simulink subsystem "queue_populator_model"  (R2020b)
settings: Solver=VariableStepAuto  StartTime=0.0  StopTime=10.0  RelTol=1e-3
undefined symbols (not defined in the file): kConsecutiveIndexDelta, kContainerIndexVector, kContainerLength, kFirstContainerIndex
libraries: move_index_lib x1
settings Model: Creator=rsub  LastModifiedBy=rsub

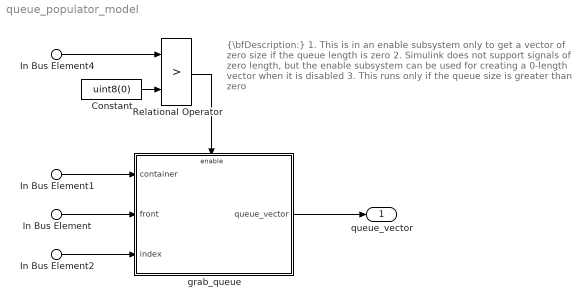
== system queue_populator_model ==
  note: {\bfDescription:}
      | 1. This is in an enable subsystem only to get a vector of zero size if the queue length is zero
      | 2. Simulink does not support signals of zero length, but the enable subsystem can be used for
      | creating a 0-length vector when it is disabled
      | 3. This runs only if the queue size is greater than zero
  In Bus Element : Inport  PortName=update_func_tx_bus  Element=front_index
  In Bus Element1 : Inport  PortName=update_func_tx_bus  Element=container_vector
  In Bus Element2 : Inport  PortName=update_func_tx_bus  Element=back_index
  In Bus Element4 : Inport  PortName=update_func_tx_bus  Element=queue_size
  Constant : Constant  Value=uint8(0)
  Relational Operator : RelationalOperator  Operator=>  OutDataTypeStr=boolean  RndMeth=Simplest
  grab_queue : Subsystem
  queue_vector : Outport
  wires:
  In Bus Element1/1 -> grab_queue/1(container)
  In Bus Element/1 -> grab_queue/2(front)
  In Bus Element2/1 -> grab_queue/3(index)
  grab_queue/1(queue_vector) -> queue_vector/1
  In Bus Element4/1 -> Relational Operator/1
  Relational Operator/1 -> grab_queue/Enable
  Constant/1 -> Relational Operator/2

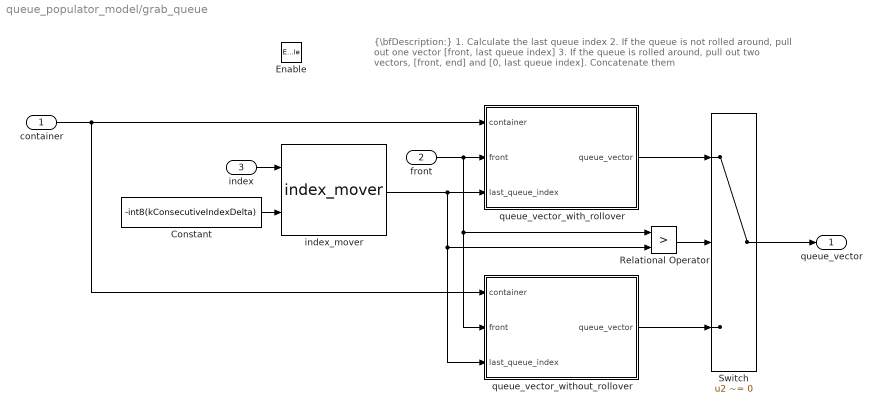
== system queue_populator_model/grab_queue ==
  note: {\bfDescription:}
      | 1. Calculate the last queue index
      | 2. If the queue is not rolled around, pull out one vector [front, last queue index]
      | 3. If the queue is rolled around, pull out two vectors, [front, end] and [0, last queue index]. Concatenate them
  container : Inport
  front : Inport  Port=2
  index : Inport  Port=3
  Enable : EnablePort  StatesWhenEnabling=reset  PropagateVarSize=During execution
  Constant : Constant  Value=-int8(kConsecutiveIndexDelta)
  Relational Operator : RelationalOperator  Operator=>  OutDataTypeStr=boolean  RndMeth=Simplest
  Switch : Switch  Criteria=u2 ~= 0  AllowDiffInputSizes=on
  index_mover : move_index_lib/index_mover  SystemSampleTime=-1  VariantActivationTime=update diagram  Latency=0  AutoFrameSizeCalculation=off
  queue_vector_with_rollover : Subsystem
  queue_vector_without_rollover : Subsystem
  queue_vector : Outport  OutputWhenDisabled=reset
  wires:
  queue_vector_with_rollover/1(queue_vector) -> Switch/1
  queue_vector_without_rollover/1(queue_vector) -> Switch/3
  container/1 -> queue_vector_with_rollover/1(container), queue_vector_without_rollover/1(container)
  index_mover/1 -> queue_vector_with_rollover/3(last_queue_index), Relational Operator/2, queue_vector_without_rollover/3(last_queue_index)
  Switch/1 -> queue_vector/1
  Relational Operator/1 -> Switch/2
  index/1 -> index_mover/1
  front/1 -> queue_vector_with_rollover/2(front), Relational Operator/1, queue_vector_without_rollover/2(front)
  Constant/1 -> index_mover/2

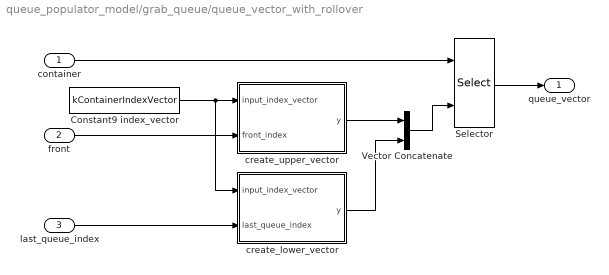
== system queue_populator_model/grab_queue/queue_vector_with_rollover ==
  container : Inport
  front : Inport  Port=2
  last_queue_index : Inport  Port=3
  Constant9 index_vector : Constant  Value=kContainerIndexVector
  Selector : Selector  IndexMode=Zero-based  InputPortWidth=kContainerLength  IndexOptions=Index vector (port)  Indices=[1 3]  OutputSizes=1
      settings: AttributesFormatString=%<IndexOptions>
  Vector Concatenate : Concatenate
  create_lower_vector : Subsystem
  create_upper_vector : Subsystem
  queue_vector : Outport
  wires:
  create_lower_vector/1(y) -> Vector Concatenate/2
  create_upper_vector/1(y) -> Vector Concatenate/1
  last_queue_index/1 -> create_lower_vector/2(last_queue_index)
  front/1 -> create_upper_vector/2(front_index)
  Constant9 index_vector/1 -> create_upper_vector/1(input_index_vector), create_lower_vector/1(input_index_vector)
  Vector Concatenate/1 -> Selector/2
  container/1 -> Selector/1
  Selector/1 -> queue_vector/1

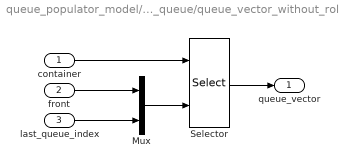
== system queue_populator_model/grab_queue/queue_vector_without_rollover ==
  container : Inport
  front : Inport  Port=2
  last_queue_index : Inport  Port=3
  Mux : Mux  Inputs=2
  Selector : Selector  IndexMode=Zero-based  InputPortWidth=kContainerLength  IndexOptions=Starting and ending indices (port)  Indices=[1 3]  OutputSizes=1
      settings: AttributesFormatString=%<IndexOptions>
  queue_vector : Outport
  wires:
  Mux/1 -> Selector/2
  last_queue_index/1 -> Mux/2
  container/1 -> Selector/1
  front/1 -> Mux/1
  Selector/1 -> queue_vector/1

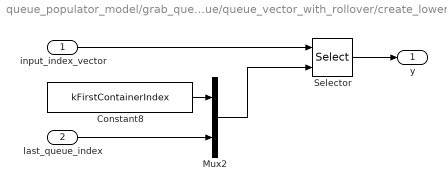
== system queue_populator_model/grab_queue/queue_vector_with_rollover/create_lower_vector ==
  input_index_vector : Inport
  last_queue_index : Inport  Port=2
  Constant8 : Constant  Value=kFirstContainerIndex
  Mux2 : Mux  Inputs=2
  Selector : Selector  IndexMode=Zero-based  InputPortWidth=kContainerLength  IndexOptions=Starting and ending indices (port)  Indices=[1 3]  OutputSizes=1
      settings: AttributesFormatString=%<IndexOptions>
  y : Outport
  wires:
  last_queue_index/1 -> Mux2/2
  Mux2/1 -> Selector/2
  Constant8/1 -> Mux2/1
  Selector/1 -> y/1
  input_index_vector/1 -> Selector/1

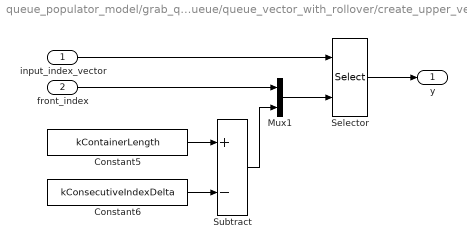
== system queue_populator_model/grab_queue/queue_vector_with_rollover/create_upper_vector ==
  input_index_vector : Inport
  front_index : Inport  Port=2
  Constant5 : Constant  Value=kContainerLength
  Constant6 : Constant  Value=kConsecutiveIndexDelta
  Mux1 : Mux  Inputs=2
  Selector : Selector  IndexMode=Zero-based  InputPortWidth=kContainerLength  IndexOptions=Starting and ending indices (port)  Indices=[1 3]  OutputSizes=1
      settings: AttributesFormatString=%<IndexOptions>
  Subtract : Sum  Inputs=+-
  y : Outport
  wires:
  Subtract/1 -> Mux1/2
  Mux1/1 -> Selector/2
  front_index/1 -> Mux1/1
  Constant5/1 -> Subtract/1
  Constant6/1 -> Subtract/2
  Selector/1 -> y/1
  input_index_vector/1 -> Selector/1
